simulink model "echo_robot_state"  (R2019a)
settings: Solver=FixedStepDiscrete  StartTime=0.0  StopTime=inf  FixedStep=0.001  RelTol=1e-3  EnableMultiTasking=on
PreLoadFcn:
  | demos_common_configs();
libraries: franka_simulink_library_misc x5, franka_simulink_library x3
settings Model: SimulationMode=external  ExtModeTrigDuration=10000  Creator=vasi_ko  LastModifiedBy=kvasios
settings DataIOCC: LimitDataPoints=on  SaveFormat=Array  ReturnWorkspaceOutputs=off
settings OptimizationCC: DefaultParameterBehavior=Inlined  EnhancedBackFolding=on  PassReuseOutputArgsAs=Individual arguments  ZeroExternalMemoryAtStartup=off  ZeroInternalMemoryAtStartup=off  OptimizeBlockOrder=speed  DifferentSizesBufferReuse=on  OptimizationCustomize=off
settings DebuggingCC: SolverPrmCheckMsg=warning  ParameterTunabilityLossMsg=error  SFUnexpectedBacktrackingDiag=warning  SFNoUnconditionalDefaultTransitionDiag=warning  SFExecutionAtInitializationDiag=none  ArithmeticOperatorsInVariantConditions=warning
settings HardwareCC: ProdBitPerLong=64  ProdHWDeviceType=Intel->x86-64 (Linux 64)  TargetBitPerLong=64  TargetBitPerPointer=64  TargetBitPerSizeT=64  TargetBitPerPtrDiffT=64  TargetLongLongMode=on  TargetIntDivRoundTo=Zero  TargetEndianess=LittleEndian  TargetWordSize=64  TargetHWDeviceType=MATLAB Host
settings ModelReferenceCC: PropagateSignalLabelsOutOfModel=off
settings SFSimCC: MATLABDynamicMemAlloc=off
settings RTWCC: SystemTargetFile=franka_emika_panda.tlc  GenCodeOnly=on  TemplateMakefile=ert_default_tmf  RTWVerbose=off  Toolchain=Franka Simulink | gmake (64-bit linux)  BuildConfiguration=Faster Runs  IncludeHyperlinkInReport=on  TargetLang=C++
settings CodeAppCC: ForceParamTrailComments=on  IgnoreCustomStorageClasses=off  OperatorAnnotations=on  SimulinkDataObjDesc=on  SFDataObjDesc=on  InsertBlockDesc=on
settings STFCustomTargetCC: TargetLangStandard=C99 (ISO)  MultiwordLength=256  GenerateSampleERTMain=on  ModelReferenceCompliant=off  CombineOutputUpdateFcns=on  ERTCustomFileBanners=on  SupportNonInlinedSFcns=off  RemoveResetFunc=on  MATLABClassNameForMDSCustomization=Simulink.SoftwareTarget.ERTCustomization  CPPClassGenCompliant=on  GRTInterface=off  UseToolchainInfoCompliant=on  SystemTargetFile=franka_emika_panda.tlc
settings ERTTargetCC: TargetLangStandard=C99 (ISO)  GenerateSampleERTMain=on  ModelReferenceCompliant=off  ParMdlRefBuildCompliant=off  CompOptLevelCompliant=off  ConcurrentExecutionCompliant=off  SupportContinuousTime=on  ModelStepFunctionPrototypeControlCompliant=off  InlinedParameterPlacement=NonHierarchical  ERTCustomFileTemplate=franka_emika_panda_file_process.tlc

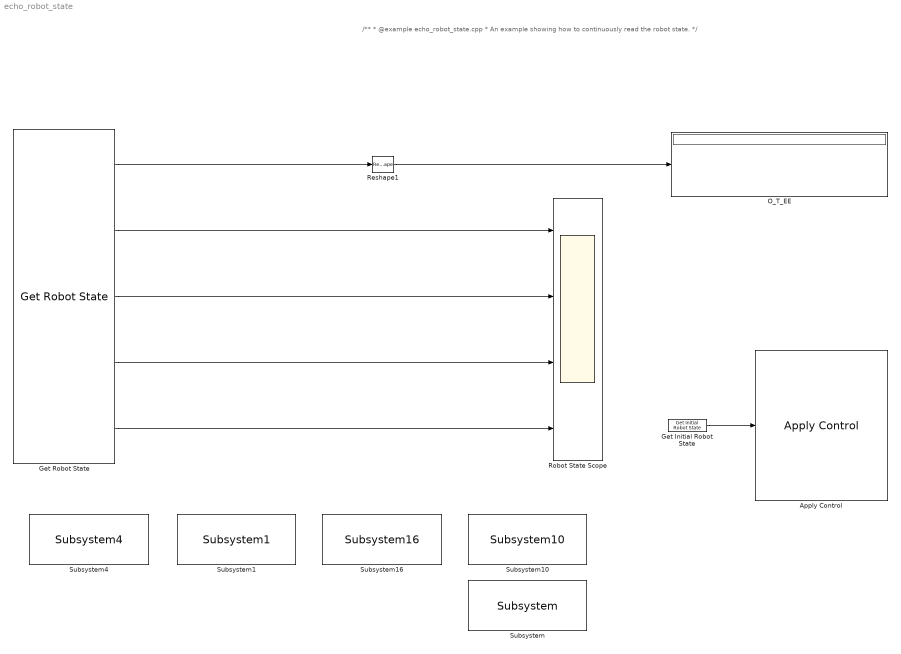
== system echo_robot_state ==
  note: /**
      |  * @example echo_robot_state.cpp
      |  * An example showing how to continuously read the robot state.
      |  */
  Apply Control : franka_simulink_library/Apply Control  robot_ip=robot_ip  gripper_attached=off  control_mode=Joint Positions - Internal Controller Mode  controller_choice=Joint Impedance Controller  elbow_control=off  collision_thresholds=100*ones(1,52)  joint_impedance=joint_impedance  cartesian_impedance=cartesian_impedance  load_inertia=load_inertia  EE_T_K=EE_T_K  init_joint_configuration_req=on  init_joint_configuration=[0, -pi/4, 0, -3 * pi/4, 0, pi/2, pi/4]
      settings: SourceProductName=Franka Emika
  Get Initial Robot State : franka_simulink_library/Get Initial Robot State  robot_ip=robot_ip  signals_requested='q_d'
      settings: SourceProductName=Franka Emika
  Get Robot State : franka_simulink_library/Get Robot State  robot_ip=robot_ip  signals_requested='O_T_EE tau_J_d tau_J K_F_ext_hat_K control_command_success_rate'
      settings: SourceProductName=Franka Emika
  O_T_EE : Display
  Reshape1 : Reshape  OutputDimensionality=Customize  OutputDimensions=[4,4]
  Robot State Scope : Scope  NumInputPorts=4
  Subsystem : franka_simulink_library_misc/Subsystem  SystemSampleTime=-1  Latency=0  AutoFrameSizeCalculation=off
  Subsystem1 : franka_simulink_library_misc/Subsystem1  SystemSampleTime=-1  Latency=0  AutoFrameSizeCalculation=off
  Subsystem10 : franka_simulink_library_misc/Subsystem10  SystemSampleTime=-1  Latency=0  AutoFrameSizeCalculation=off
  Subsystem16 : franka_simulink_library_misc/Subsystem16  SystemSampleTime=-1  Latency=0  AutoFrameSizeCalculation=off
  Subsystem4 : franka_simulink_library_misc/Subsystem4  SystemSampleTime=-1  Latency=0  AutoFrameSizeCalculation=off
  wires:
  Reshape1/1 -> O_T_EE/1
  Get Robot State/1 -> Reshape1/1
  Get Robot State/3 -> Robot State Scope/2
  Get Robot State/2 -> Robot State Scope/1
  Get Robot State/4 -> Robot State Scope/3
  Get Robot State/5 -> Robot State Scope/4
  Get Initial Robot State/1 -> Apply Control/1
